simulink model "quart_vehicule_suspension_active"  (R2018a)
settings: Solver=VariableStepAuto  StartTime=0.0  StopTime=10.0  RelTol=1e-3
settings Model: Creator=hp  LastModifiedBy=hp

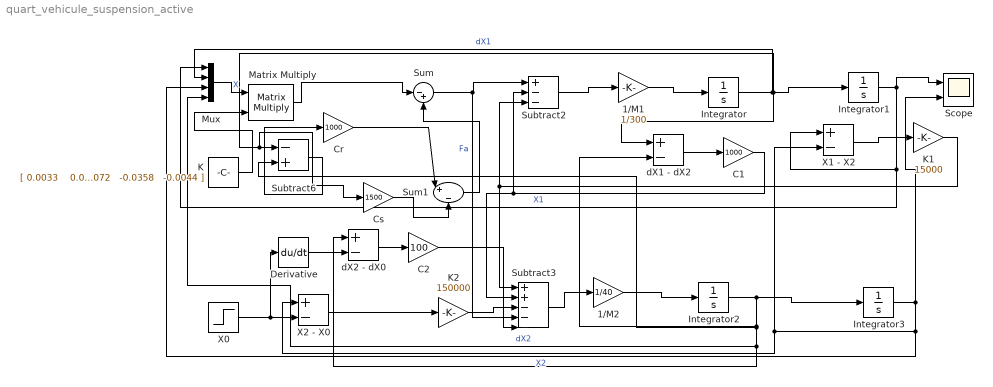
== system quart_vehicule_suspension_active ==
  1/M1 : Gain  Gain=1/300
  1/M2 : Gain  Gain=1/40
  C1 : Gain  Gain=1000
  C2 : Gain  Gain=100
  Cr : Gain  Gain=1000
  Cs : Gain  Gain=1500
  Derivative : Derivative
  Integrator{,1..3} (4 alike) : Integrator
  K : Constant  Value=|
      | [ 0.0033    0.0072   -0.0358   -0.0044
      | ]
  K1 : Gain  Gain=15000
  K2 : Gain  Gain=150000
  Matrix Multiply : Product  Multiplication=Matrix(*)
  Mux : Mux
  Scope : Scope  NumInputPorts=2
  Subtract2 : Sum  Inputs=+--
  Subtract3 : Sum  Inputs=|+|+|-|-|-
  Subtract6 : Sum  Inputs=-+
  Sum : Sum  Inputs=|-+
  Sum1 : Sum  Inputs=|+|-
  X0 : Step  After=0.05  SampleTime=0
  X1 - X2 : Sum  Inputs=+-
  X2 - X0 : Sum  Inputs=+-
  dX1 - dX2 : Sum  Inputs=+-
  dX2 - dX0 : Sum  Inputs=+-
  wires:
  C2/1 -> Subtract3/5
  Derivative/1 -> dX2 - dX0/2
  Integrator1/1 -> Mux/1, X1 - X2/1, Scope/1  "X1"
  dX2 - dX0/1 -> C2/1
  X2 - X0/1 -> K2/1
  Subtract2/1 -> 1/M1/1
  X0/1 -> Derivative/1, X2 - X0/2
  C1/1 -> Subtract3/2, Subtract2/2
  X1 - X2/1 -> K1/1
  Integrator3/1 -> Mux/3, X2 - X0/1, X1 - X2/2, Scope/2  "X2"
  1/M1/1 -> Integrator/1
  dX1 - dX2/1 -> C1/1
  Integrator/1 -> Mux/2, dX1 - dX2/1, Integrator1/1, Cs/1, Subtract6/1  "dX1"
  Integrator2/1 -> Subtract6/2, Mux/4, dX2 - dX0/1, dX1 - dX2/2, Integrator3/1  "dX2"
  Subtract3/1 -> 1/M2/1
  1/M2/1 -> Integrator2/1
  K2/1 -> Subtract3/3
  K1/1 -> Subtract3/1, Subtract2/3
  Matrix Multiply/1 -> Sum/1
  Mux/1 -> Matrix Multiply/1  "X"
  K/1 -> Matrix Multiply/2
  Sum/1 -> Subtract3/4, Subtract2/1  "Fa"
  Cs/1 -> Sum1/2
  Subtract6/1 -> Cr/1
  Cr/1 -> Sum1/1
  Sum1/1 -> Sum/2
